simulink model "cel_sim"  (R2020a)
settings: Solver=VariableStepAuto  StartTime=0.0  StopTime=t_sim  MaxStep=0.1  RelTol=1e-3
undefined symbols (not defined in the file): B_cel0, E_cel0, v0, x0, y0, z0
libraries: simulink x3
settings Model: Creator=RAFAL  LastModifiedBy=rafal
settings DebuggingCC: ArtificialAlgebraicLoopMsg=none

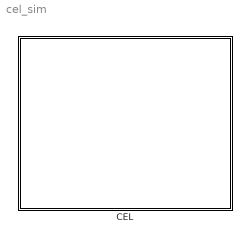
== system cel_sim ==
  CEL : Subsystem

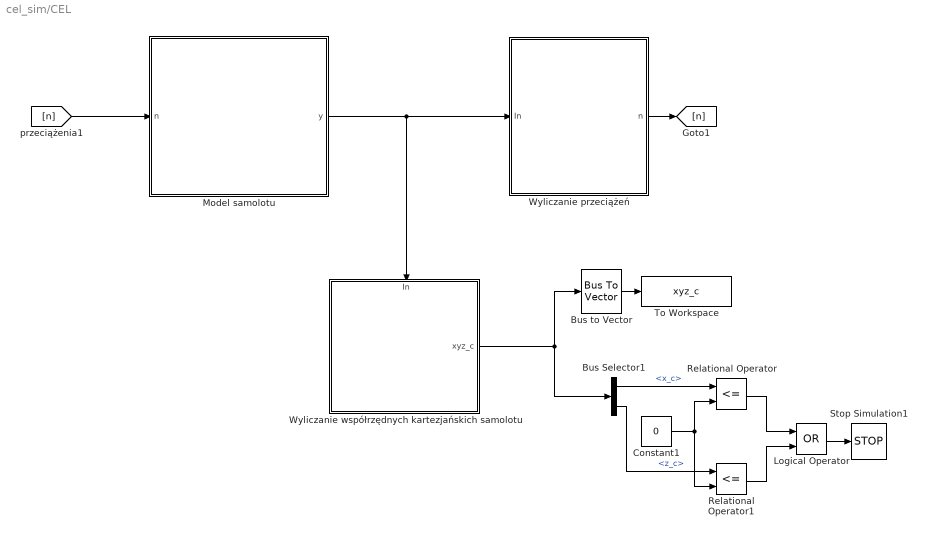
== system cel_sim/CEL ==
  Bus Selector1 : BusSelector  OutputSignals=x_c,z_c
  Bus to Vector : BusToVector
  Constant1 : Constant  Value=0
  Logical Operator : Logic  Operator=OR  AllPortsSameDT=off  OutDataTypeStr=boolean
  Model samolotu : Subsystem
  Relational Operator : RelationalOperator  Operator=<=  OutDataTypeStr=boolean  RndMeth=Simplest
  Relational Operator1 : RelationalOperator  Operator=<=  OutDataTypeStr=boolean  RndMeth=Simplest
  Stop Simulation1 : Stop
  To Workspace : ToWorkspace  VariableName=xyz_c  SaveFormat=Timeseries  SampleTime=0.25
  Wyliczanie przeciążeń : Subsystem
  Wyliczanie współrzędnych kartezjańskich samolotu : Subsystem
      settings: PortSchema="{\"entries\":[{\"content\":{\"sides\":[{\"content\":{\"connectorIds\":[]},\"type\":\"ConnectorPlacement.EquallySpacedRectSide\",\"uuid\":\"2ae1aec2-e4bf-4b19-9a5e-448bf8307686\"},{\"content\":{\"connectorIds\":[\"Out1\"],\"side\":\"RIGHT\"},\"type\":\"ConnectorPlacement.EquallySpacedRectSide\",\"uuid\":\"06d750e3-693c-429f-872d-17e0894ecc7b\"},{\"content\":{\"connectorIds\":[\"In1\"],\"side\":\"TOP\"},\"type\":\"ConnectorPlacement.EquallySpacedRectSide\",\"uuid\":\"7749f68d-516b-452e-a489-1265694a2423\"}]},\"type\":\"ConnectorPlacement.EquallySpacedConnector\",\"uuid\":\"3f3251d9-794b-41fb-a72e-7606b000567a\"}],\"packageUris\":[\"http://schema.mathworks.com/mf0/Connector/19700101\"],\"version\":\"1.0\"}"
  wires:
  Relational Operator/1 -> Logical Operator/1
  Constant1/1 -> Relational Operator1/2, Relational Operator/2
  Wyliczanie współrzędnych kartezjańskich samolotu/1(xyz_c) -> Bus to Vector/1, Bus Selector1/1
  Wyliczanie przeciążeń/1(n) -> [n]
  Bus Selector1/1 -> Relational Operator/1  "<x_c>"
  Bus Selector1/2 -> Relational Operator1/1  "<z_c>"
  Relational Operator1/1 -> Logical Operator/2
  Logical Operator/1 -> Stop Simulation1/1
  Bus to Vector/1 -> To Workspace/1
  Model samolotu/1(y) -> Wyliczanie przeciążeń/1(In), Wyliczanie współrzędnych kartezjańskich samolotu/1(In)
  [n] -> Model samolotu/1(n)

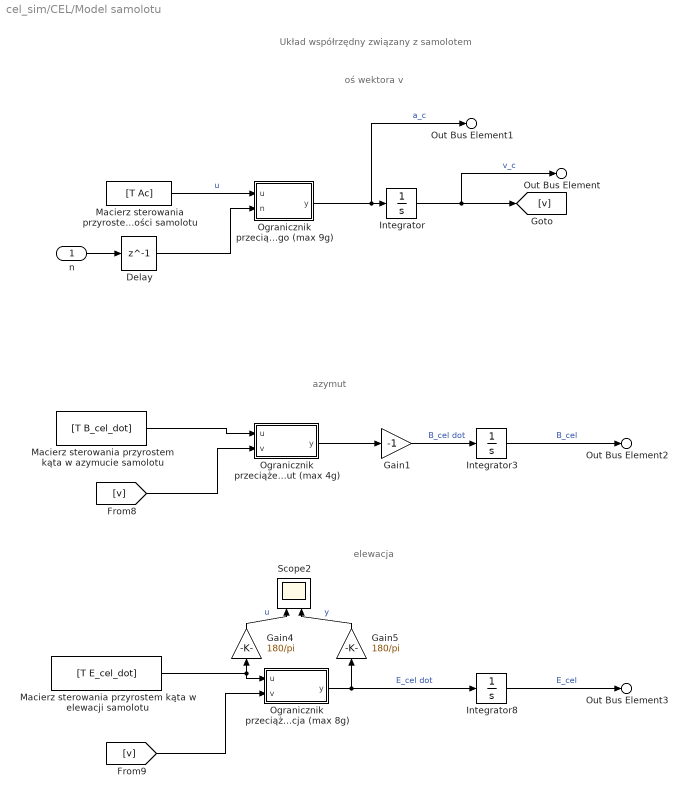
== system cel_sim/CEL/Model samolotu ==
  note: Układ współrzędny związany z samolotem
  note: oś wektora v
  note: elewacja
  note: azymut
  n : Inport
  Delay : Delay  DelayLength=1
  Gain1 : Gain  Gain=-1
  Gain4 : Gain  Gain=180/pi
  Gain5 : Gain  Gain=180/pi
  Integrator : Integrator  InitialCondition=v0
  Integrator3 : Integrator  InitialCondition=B_cel0
  Integrator8 : Integrator  InitialCondition=E_cel0
  Macierz sterowania przyrostem kąta w azymucie samolotu : FromWorkspace  VariableName=[T B_cel_dot]
  Macierz sterowania przyrostem kąta w elewacji samolotu : FromWorkspace  VariableName=[T E_cel_dot]
  "Macierz sterowania przyrostem prędkości samolotu " : FromWorkspace  VariableName=[T Ac]
  Ogranicznik przeciążenia wypadkowego (max 9g) : Subsystem
  Ogranicznik przeciążenia azymut (max 4g) : Subsystem
  Ogranicznik przeciążenia elewacja (max 8g) : Subsystem
  Scope2 : Scope  NumInputPorts=2
  Out Bus Element : Outport  PortName=y  Element=v_c
  Out Bus Element1 : Outport  PortName=y  Element=a_c
  Out Bus Element2 : Outport  PortName=y  Element=B_cel
  Out Bus Element3 : Outport  PortName=y  Element=E_cel
  wires:
  Macierz sterowania przyrostem kąta w azymucie samolotu/1 -> Ogranicznik przeciążenia azymut (max 4g)/1(u)
  Ogranicznik przeciążenia elewacja (max 8g)/1(y) -> Gain5/1, Integrator8/1  "E_cel dot"
  Integrator/1 -> Out Bus Element/1, [v]  "v_c"
  Macierz sterowania przyrostem kąta w elewacji samolotu/1 -> Ogranicznik przeciążenia elewacja (max 8g)/1(u), Gain4/1
  Ogranicznik przeciążenia wypadkowego (max 9g)/1(y) -> Out Bus Element1/1, Integrator/1  "a_c"
  [v] -> Ogranicznik przeciążenia elewacja (max 8g)/2(v)
  Ogranicznik przeciążenia azymut (max 4g)/1(y) -> Gain1/1
  [v] -> Ogranicznik przeciążenia azymut (max 4g)/2(v)
  Gain1/1 -> Integrator3/1  "B_cel dot"
  "Macierz sterowania przyrostem prędkości samolotu "/1 -> Ogranicznik przeciążenia wypadkowego (max 9g)/1(u)  "u"
  Integrator3/1 -> Out Bus Element2/1  "B_cel"
  Integrator8/1 -> Out Bus Element3/1  "E_cel"
  Gain4/1 -> Scope2/1  "u"
  Gain5/1 -> Scope2/2  "y"
  n/1 -> Delay/1
  Delay/1 -> Ogranicznik przeciążenia wypadkowego (max 9g)/2(n)

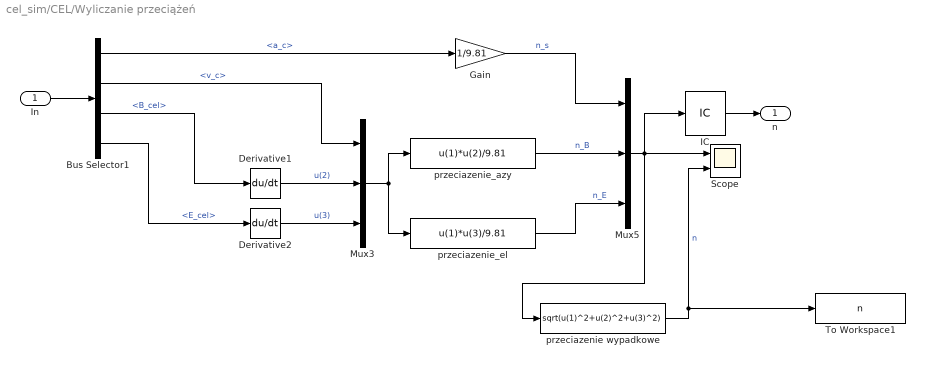
== system cel_sim/CEL/Wyliczanie przeciążeń ==
  In : Inport
  Bus Selector1 : BusSelector  OutputSignals=a_c,v_c,B_cel,E_cel
  Derivative1 : Derivative
  Derivative2 : Derivative
  Gain : Gain  Gain=1/9.81
  IC : InitialCondition  Value=0
  Mux3 : Mux  Inputs=3
  Mux5 : Mux  Inputs=3
  Scope : Scope  NumInputPorts=2
  To Workspace1 : ToWorkspace  VariableName=n  SaveFormat=Timeseries  SampleTime=0.25
  przeciazenie wypadkowe : Fcn  Expr=sqrt(u(1)^2+u(2)^2+u(3)^2)
  przeciazenie_azy : Fcn  Expr=u(1)*u(2)/9.81
  przeciazenie_el : Fcn  Expr=u(1)*u(3)/9.81
  n : Outport
  wires:
  Derivative2/1 -> Mux3/3  "u(3)"
  Mux3/1 -> przeciazenie_azy/1, przeciazenie_el/1
  przeciazenie wypadkowe/1 -> Scope/2, To Workspace1/1  "n"
  przeciazenie_azy/1 -> Mux5/2  "n_B"
  przeciazenie_el/1 -> Mux5/3  "n_E"
  Bus Selector1/4 -> Derivative2/1  "<E_cel>"
  Gain/1 -> Mux5/1  "n_s"
  Bus Selector1/3 -> Derivative1/1  "<B_cel>"
  Bus Selector1/2 -> Mux3/1  "<v_c>"
  Derivative1/1 -> Mux3/2  "u(2)"
  In/1 -> Bus Selector1/1
  Bus Selector1/1 -> Gain/1  "<a_c>"
  Mux5/1 -> IC/1, Scope/1, przeciazenie wypadkowe/1
  IC/1 -> n/1

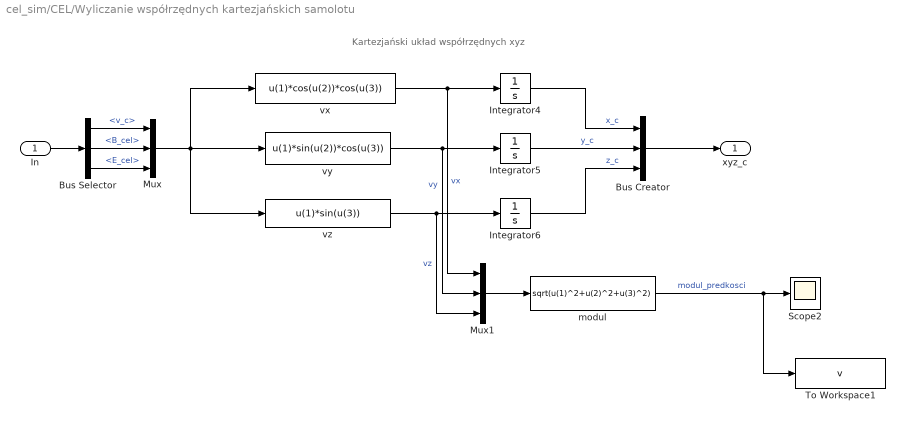
== system cel_sim/CEL/Wyliczanie współrzędnych kartezjańskich samolotu ==
  note: Kartezjański układ współrzędnych xyz
  In : Inport
  Bus Creator : BusCreator  Inputs=3
  Bus Selector : BusSelector  OutputSignals=v_c,B_cel,E_cel
  Integrator4 : Integrator  InitialCondition=x0
  Integrator5 : Integrator  InitialCondition=y0
  Integrator6 : Integrator  InitialCondition=z0
  Mux : Mux  Inputs=3
  Mux1 : Mux  Inputs=3
  Scope2 : Scope
  To Workspace1 : ToWorkspace  VariableName=v  SaveFormat=Timeseries  SampleTime=0.25
  modul : Fcn  Expr=sqrt(u(1)^2+u(2)^2+u(3)^2)
  vx : Fcn  Expr=u(1)*cos(u(2))*cos(u(3))
  vy : Fcn  Expr=u(1)*sin(u(2))*cos(u(3))
  vz : Fcn  Expr=u(1)*sin(u(3))
  xyz_c : Outport
  wires:
  vy/1 -> Integrator5/1, Mux1/2  "vy"
  Mux1/1 -> modul/1
  vz/1 -> Mux1/3, Integrator6/1  "vz"
  modul/1 -> To Workspace1/1, Scope2/1  "modul_predkosci"
  vx/1 -> Mux1/1, Integrator4/1  "vx"
  Bus Creator/1 -> xyz_c/1
  Integrator6/1 -> Bus Creator/3  "z_c"
  Integrator5/1 -> Bus Creator/2  "y_c"
  Integrator4/1 -> Bus Creator/1  "x_c"
  In/1 -> Bus Selector/1
  Mux/1 -> vz/1, vy/1, vx/1
  Bus Selector/1 -> Mux/1  "<v_c>"
  Bus Selector/2 -> Mux/2  "<B_cel>"
  Bus Selector/3 -> Mux/3  "<E_cel>"

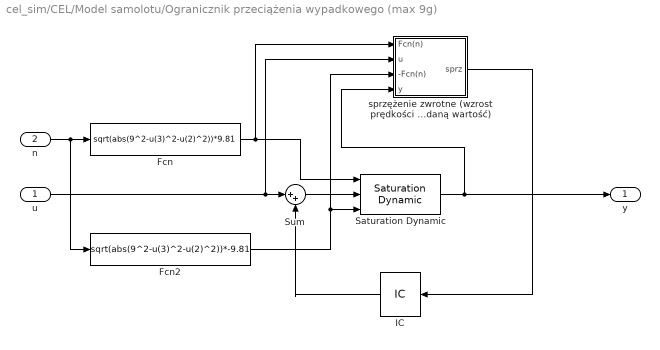
== system cel_sim/CEL/Model samolotu/Ogranicznik przeciążenia wypadkowego (max 9g) ==
  u : Inport
  n : Inport  Port=2
  Fcn : Fcn  Expr=sqrt(abs(9^2-u(3)^2-u(2)^2))*9.81
  Fcn2 : Fcn  Expr=sqrt(abs(9^2-u(3)^2-u(2)^2))*-9.81
  IC : InitialCondition  Value=0
  Saturation Dynamic : simulink/Discontinuities/Saturation Dynamic  OutMin=[]  OutMax=[]  OutDataTypeStr=Inherit: Same as second input  OutDataType=fixdt(1, 16)  OutScaling=2^-10  DoSatur=off
  Sum : Sum  Inputs=|++
  sprzężenie zwrotne (wzrost prędkości o zadaną wartość) : Subsystem
  y : Outport
  wires:
  n/1 -> Fcn2/1, Fcn/1
  Fcn2/1 -> sprzężenie zwrotne (wzrost prędkości o zadaną wartość)/3(-Fcn(n)), Saturation Dynamic/3
  Saturation Dynamic/1 -> sprzężenie zwrotne (wzrost prędkości o zadaną wartość)/4(y), y/1
  sprzężenie zwrotne (wzrost prędkości o zadaną wartość)/1(sprz) -> IC/1
  u/1 -> sprzężenie zwrotne (wzrost prędkości o zadaną wartość)/2(u), Sum/1
  Sum/1 -> Saturation Dynamic/2
  Fcn/1 -> sprzężenie zwrotne (wzrost prędkości o zadaną wartość)/1(Fcn(n)), Saturation Dynamic/1
  IC/1 -> Sum/2

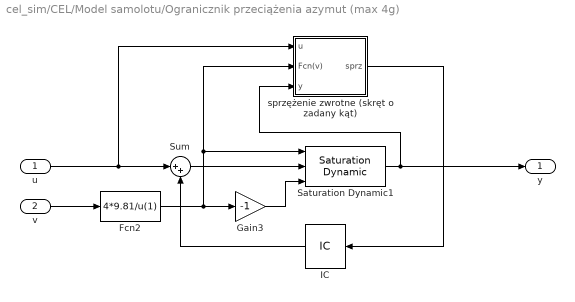
== system cel_sim/CEL/Model samolotu/Ogranicznik przeciążenia azymut (max 4g) ==
  u : Inport
  v : Inport  Port=2
  Fcn2 : Fcn  Expr=4*9.81/u(1)
  Gain3 : Gain  Gain=-1
  IC : InitialCondition  Value=0
  Saturation Dynamic1 : simulink/Discontinuities/Saturation Dynamic  OutMin=[]  OutMax=[]  OutDataTypeStr=Inherit: Same as second input  OutDataType=fixdt(1, 16)  OutScaling=2^-10  DoSatur=off
  Sum : Sum  Inputs=|++
  sprzężenie zwrotne (skręt o zadany kąt) : Subsystem
  y : Outport
  wires:
  v/1 -> Fcn2/1
  Gain3/1 -> Saturation Dynamic1/3
  Saturation Dynamic1/1 -> sprzężenie zwrotne (skręt o zadany kąt)/3(y), y/1
  Sum/1 -> Saturation Dynamic1/2
  u/1 -> sprzężenie zwrotne (skręt o zadany kąt)/1(u), Sum/1
  Fcn2/1 -> sprzężenie zwrotne (skręt o zadany kąt)/2(Fcn(v)), Saturation Dynamic1/1, Gain3/1
  sprzężenie zwrotne (skręt o zadany kąt)/1(sprz) -> IC/1
  IC/1 -> Sum/2

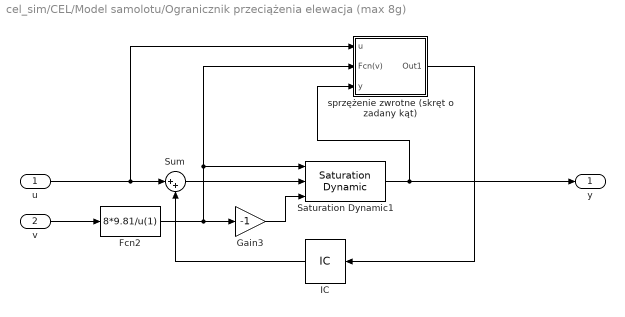
== system cel_sim/CEL/Model samolotu/Ogranicznik przeciążenia elewacja (max 8g) ==
  u : Inport
  v : Inport  Port=2
  Fcn2 : Fcn  Expr=8*9.81/u(1)
  Gain3 : Gain  Gain=-1
  IC : InitialCondition  Value=0
  Saturation Dynamic1 : simulink/Discontinuities/Saturation Dynamic  OutMin=[]  OutMax=[]  OutDataTypeStr=Inherit: Same as second input  OutDataType=fixdt(1, 16)  OutScaling=2^-10  DoSatur=off
  Sum : Sum  Inputs=|++
  sprzężenie zwrotne (skręt o zadany kąt) : Subsystem
  y : Outport
  wires:
  Gain3/1 -> Saturation Dynamic1/3
  v/1 -> Fcn2/1
  u/1 -> sprzężenie zwrotne (skręt o zadany kąt)/1(u), Sum/1
  Saturation Dynamic1/1 -> sprzężenie zwrotne (skręt o zadany kąt)/3(y), y/1
  Sum/1 -> Saturation Dynamic1/2
  Fcn2/1 -> sprzężenie zwrotne (skręt o zadany kąt)/2(Fcn(v)), Saturation Dynamic1/1, Gain3/1
  sprzężenie zwrotne (skręt o zadany kąt)/1(Out1) -> IC/1
  IC/1 -> Sum/2

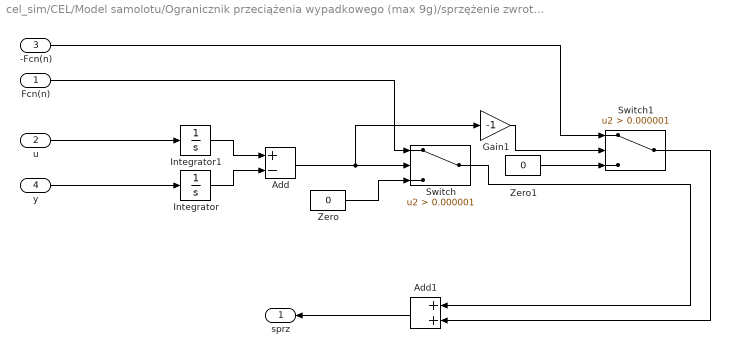
== system cel_sim/CEL/Model samolotu/Ogranicznik przeciążenia wypadkowego (max 9g)/sprzężenie zwrotne (wzrost prędkości o zadaną wartość) ==
  Fcn(n) : Inport
  u : Inport  Port=2
  -Fcn(n) : Inport  Port=3
  y : Inport  Port=4
  Add : Sum  Inputs=+-
  Add1 : Sum
  Gain1 : Gain  Gain=-1
  Integrator : Integrator
  Integrator1 : Integrator
  Switch : Switch  Criteria=u2 > Threshold  Threshold=0.000001
  Switch1 : Switch  Criteria=u2 > Threshold  Threshold=0.000001
  Zero : Constant  Value=0  OutDataTypeStr=Inherit: Inherit via back propagation
  Zero1 : Constant  Value=0  OutDataTypeStr=Inherit: Inherit via back propagation
  sprz : Outport
  wires:
  Integrator/1 -> Add/2
  Add/1 -> Gain1/1, Switch/2
  Zero/1 -> Switch/3
  Integrator1/1 -> Add/1
  Gain1/1 -> Switch1/2
  Zero1/1 -> Switch1/3
  Switch/1 -> Add1/1
  Switch1/1 -> Add1/2
  Fcn(n)/1 -> Switch/1
  u/1 -> Integrator1/1
  y/1 -> Integrator/1
  Add1/1 -> sprz/1
  -Fcn(n)/1 -> Switch1/1

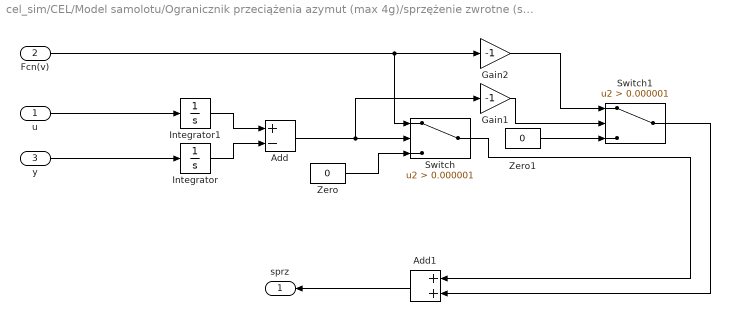
== system cel_sim/CEL/Model samolotu/Ogranicznik przeciążenia azymut (max 4g)/sprzężenie zwrotne (skręt o zadany kąt) ==
  u : Inport
  Fcn(v) : Inport  Port=2
  y : Inport  Port=3
  Add : Sum  Inputs=+-
  Add1 : Sum
  Gain1 : Gain  Gain=-1
  Gain2 : Gain  Gain=-1
  Integrator : Integrator
  Integrator1 : Integrator
  Switch : Switch  Criteria=u2 > Threshold  Threshold=0.000001
  Switch1 : Switch  Criteria=u2 > Threshold  Threshold=0.000001
  Zero : Constant  Value=0  OutDataTypeStr=Inherit: Inherit via back propagation
  Zero1 : Constant  Value=0  OutDataTypeStr=Inherit: Inherit via back propagation
  sprz : Outport
  wires:
  Integrator/1 -> Add/2
  Add/1 -> Gain1/1, Switch/2
  Zero/1 -> Switch/3
  Integrator1/1 -> Add/1
  Gain1/1 -> Switch1/2
  Zero1/1 -> Switch1/3
  Switch/1 -> Add1/1
  Gain2/1 -> Switch1/1
  Switch1/1 -> Add1/2
  Fcn(v)/1 -> Switch/1, Gain2/1
  u/1 -> Integrator1/1
  y/1 -> Integrator/1
  Add1/1 -> sprz/1

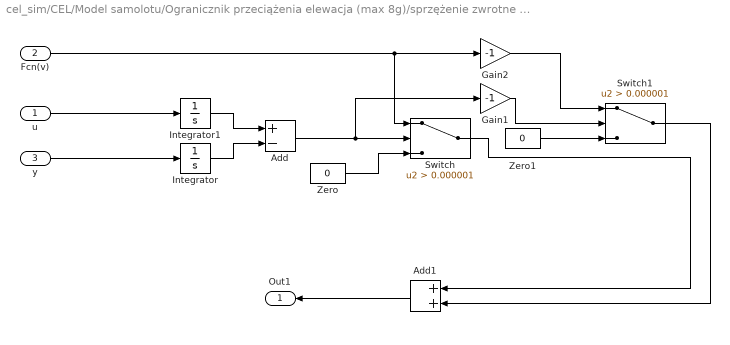
== system cel_sim/CEL/Model samolotu/Ogranicznik przeciążenia elewacja (max 8g)/sprzężenie zwrotne (skręt o zadany kąt) ==
  u : Inport
  Fcn(v) : Inport  Port=2
  y : Inport  Port=3
  Add : Sum  Inputs=+-
  Add1 : Sum
  Gain1 : Gain  Gain=-1
  Gain2 : Gain  Gain=-1
  Integrator : Integrator
  Integrator1 : Integrator
  Switch : Switch  Criteria=u2 > Threshold  Threshold=0.000001
  Switch1 : Switch  Criteria=u2 > Threshold  Threshold=0.000001
  Zero : Constant  Value=0  OutDataTypeStr=Inherit: Inherit via back propagation
  Zero1 : Constant  Value=0  OutDataTypeStr=Inherit: Inherit via back propagation
  Out1 : Outport
  wires:
  Integrator/1 -> Add/2
  Add/1 -> Gain1/1, Switch/2
  Zero/1 -> Switch/3
  Integrator1/1 -> Add/1
  Gain1/1 -> Switch1/2
  Zero1/1 -> Switch1/3
  Switch/1 -> Add1/1
  Gain2/1 -> Switch1/1
  Switch1/1 -> Add1/2
  Fcn(v)/1 -> Switch/1, Gain2/1
  u/1 -> Integrator1/1
  y/1 -> Integrator/1
  Add1/1 -> Out1/1
